simulink model "SWC_HALOUT_type"  (R2021b)
settings: Solver=FixedStepDiscrete  StartTime=0.0  StopTime=10.0  FixedStep=0.005  RelTol=1e-3
undefined symbols (not defined in the file): DIDLen_APPD, DIDLen_APPE, DIDLen_APPPedalZP, DIDLen_APSFunConfig, DIDLen_AutoLock, DIDLen_AutoWipHSpdEN, DIDLen_CALID, DIDLen_CDEODT, DIDLen_CLRDIST, DIDLen_DKCBLESta, DIDLen_DKCKey, DIDLen_DKCSta, DIDLen_DoorNFCAnchorSta, DIDLen_DRLDis, DIDLen_DynoMode, DIDLen_ECUNAME, DIDLen_FDDKCCoordXY, DIDLen_FMHTimer, DIDLen_LFLowPresThre, DIDLen_LFSensorID, DIDLen_LIDAAnchorSta, DIDLen_LRLowPresThre, DIDLen_LRSensorID, DIDLen_MILDIST, DIDLen_NUMPSATRIPSFLTMEMCLR, DIDLen_NVMPedalZP, DIDLen_OBDReq, DIDLen_ODOMETER, DIDLen_PKE, DIDLen_ProtocolId, DIDLen_PSA, DIDLen_QTYPSATRIPS, DIDLen_RFLowPresThre, DIDLen_RFSensorID, DIDLen_RRLowPresThre, DIDLen_RRSensorID, DIDLen_RUNTM, DIDLen_SensorMode, DIDLen_TestGroup, DIDLen_TireSize, DIDLen_TPMSLearnSta, DIDLen_TurnLampFLThreCurr, DIDLen_TurnLampFRThreCurr, DIDLen_TurnLampRLThreCurr, DIDLen_TurnLampRRThreCurr, DIDLen_UIDSta, DIDLen_USSConfig, DIDLen_UWBAnchorSta, DIDLen_VIN, DIDLen_VSS, DIDLen_WhlPres, DIDLen_WhlSensorBattSta, DIDLen_WhlTmp, DIDLen_WipRLSCmdCutFilter, DIDLen_WipRLSCmdHoldFilter, DIDLen_XWDMode, DIDNum_APPD, DIDNum_APPE, DIDNum_APPPedalZP, DIDNum_APSFunConfig ... (+504)
libraries: simulink x893, FVT_lib x320, hdlsllib x6, hcu_lib x5, halout x1
(part 1 of 11)
settings Model: DataDictionary=APPTypes.sldd  Creator=FVT23010  LastModifiedBy=FVT23033
settings DataIOCC: SaveFormat=StructureWithTime
settings OptimizationCC: DefaultParameterBehavior=Inlined  EnhancedBackFolding=on  PassReuseOutputArgsAs=Individual arguments  ZeroExternalMemoryAtStartup=off  ZeroInternalMemoryAtStartup=off  OptimizeBlockOrder=speed  DifferentSizesBufferReuse=on  OptimizationCustomize=off  EfficientTunableParamExpr=on
settings DebuggingCC: ParameterTunabilityLossMsg=error
settings HardwareCC: ProdBitPerPointer=32  ProdBitPerSizeT=32  ProdBitPerPtrDiffT=32  ProdLargestAtomicInteger=Long  ProdLargestAtomicFloat=Double  ProdWordSize=32  ProdLongLongMode=on  ProdHWDeviceType=ARM Compatible->ARM Cortex-M
settings ModelReferenceCC: ModelReferenceNumInstancesAllowed=Single
settings SFSimCC: MATLABDynamicMemAlloc=off
settings RTWCC: Description=AUTOSAR  SystemTargetFile=autosar.tlc  GenCodeOnly=on  TemplateMakefile=ert_default_tmf  PortableWordSizes=on
settings CodeAppCC: ForceParamTrailComments=on  IgnoreCustomStorageClasses=off  OperatorAnnotations=on  SimulinkDataObjDesc=on  SFDataObjDesc=on  InsertBlockDesc=on
settings STFCustomTargetCC: TargetLangStandard=C99 (ISO)  UtilityFuncGeneration=Shared location  MultiwordLength=256  ParMdlRefBuildCompliant=on  CompOptLevelCompliant=on  IncludeMdlTerminateFcn=off  CombineOutputUpdateFcns=on  SuppressErrorStatus=on  ERTCustomFileBanners=on  SupportNonFinite=off  SupportComplex=off  SupportContinuousTime=off  SupportNonInlinedSFcns=off  RemoveResetFunc=on  MATLABClassNameForMDSCustomization=Simulink.SoftwareTarget.ERTCustomization  AutosarCompliant=on  GRTInterface=off  UseToolchainInfoCompliant=on  GenerateSharedConstants=off  LookupTableObjectStructAxisOrder=2,1,3,4,...  LUTObjectStructOrderEvenSpacing=Size,Table,Breakpoints  SystemTargetFile=autosar.tlc
settings ERTTargetCC: TargetLangStandard=C99 (ISO)  UtilityFuncGeneration=Shared location  ConcurrentExecutionCompliant=off  IncludeMdlTerminateFcn=off  SuppressErrorStatus=on  SupportNonFinite=off  SupportComplex=off  ModelStepFunctionPrototypeControlCompliant=off  CPPClassGenCompliant=off  AutosarCompliant=on  GenerateSharedConstants=off  LookupTableObjectStructAxisOrder=2,1,3,4,...  LUTObjectStructOrderEvenSpacing=Size,Table,Breakpoints  GenerateASAP2=on  InlinedParameterPlacement=NonHierarchical  ERTCustomFileTemplate=example_file_process.tlc  ConvertIfToSwitch=off  SuppressUnreachableDefaultCases=off  BooleanTrueId=true_MatlabRTW  BooleanFalseId=false_MatlabRTW

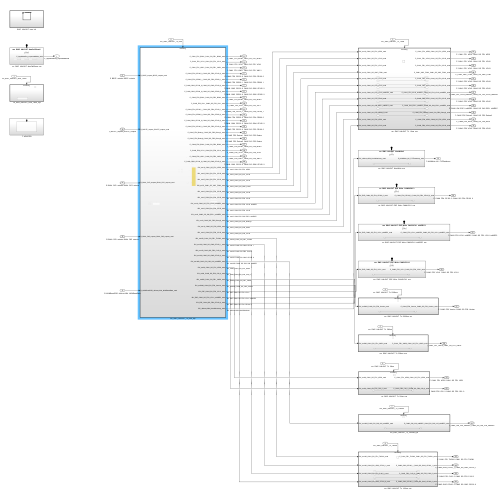
[thumbnail: Simulink's stored preview of the top-level diagram]
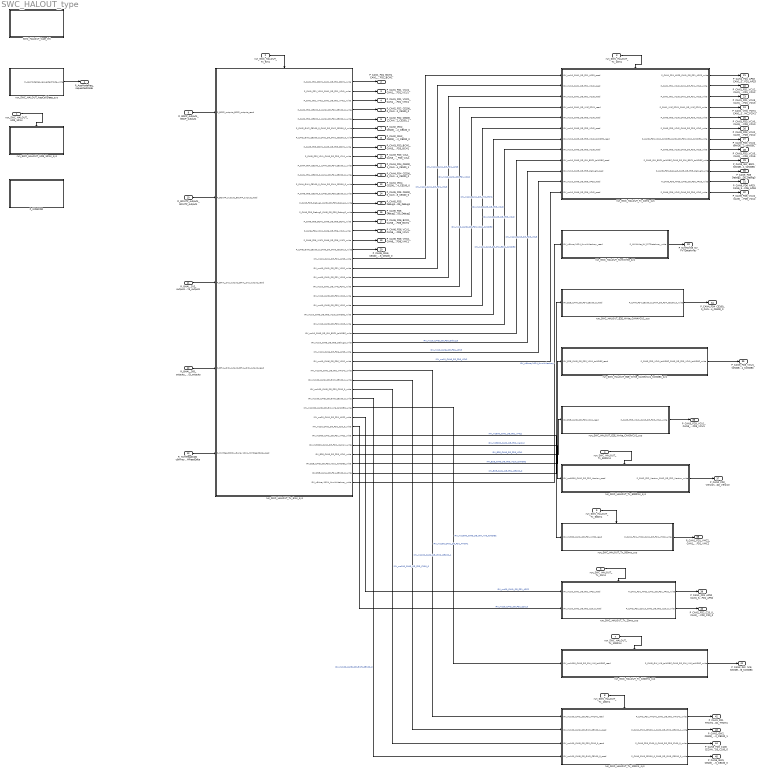
== system SWC_HALOUT_type ==
  run_SWC_HALOUT_UDS_10ms : Inport  SampleTime=0.01  OutputFunctionCall=on
  run_SWC_HALOUT_Tx_5ms : Inport  Port=2  SampleTime=0.005  OutputFunctionCall=on
  run_SWC_HALOUT_Tx_10ms : Inport  Port=3  SampleTime=0.01  OutputFunctionCall=on
  run_SWC_HALOUT_Tx_5000ms : Inport  Port=4  SampleTime=5  OutputFunctionCall=on
  run_SWC_HALOUT_Tx_500ms : Inport  Port=5  SampleTime=0.5  OutputFunctionCall=on
  run_SWC_HALOUT_Tx_20ms : Inport  Port=6  SampleTime=0.02  OutputFunctionCall=on
  run_SWC_HALOUT_Tx_1000ms : Inport  Port=7  SampleTime=1  OutputFunctionCall=on
  run_SWC_HALOUT_Tx_100ms : Inport  Port=8  SampleTime=0.1  OutputFunctionCall=on
  R_BSCP_outputs_BSCP_outputs : Inport  Port=9  OutDataTypeStr=Bus: BSCP_outputs  PortDimensions=1  BusOutputAsStruct=on
  R_BOUTP_outputs_BOUTP_outputs : Inport  Port=10  OutDataTypeStr=Bus: BOUTP_outputs  PortDimensions=1  BusOutputAsStruct=on
  R_BHAL_SYS_outputs_BHAL_SYS_outputs : Inport  Port=11  OutDataTypeStr=Bus: BHAL_SYS_outputs  PortDimensions=1  BusOutputAsStruct=on
  R_BHAL_DID_outputs_BHAL_DID_outputs : Inport  Port=12  OutDataTypeStr=Bus: BHAL_DID_outputs  PortDimensions=1  BusOutputAsStruct=on
  R_NVMReadCDD_u8Array1024_NVMReadData : Inport  Port=13  OutDataTypeStr=uint8  PortDimensions=1024
  P_WDGCDD : Subsystem
  SWC_HALOUT_type_Init : Subsystem
  run_SWC_HALOUT_AppCallSleep_sys : Subsystem
  run_SWC_HALOUT_E2E_Write_CAN3VCU1_sys : Subsystem
  run_SWC_HALOUT_E2E_Write_CAN3VCU1_toNIDEC_sys : Subsystem
  run_SWC_HALOUT_E2E_Write_CAN4VCU1_sys : Subsystem
  run_SWC_HALOUT_NvmWrite_sys : Subsystem
  run_SWC_HALOUT_Tx_1000ms_sys : Subsystem
  run_SWC_HALOUT_Tx_100ms_sys : Subsystem
  run_SWC_HALOUT_Tx_10ms_sys : Subsystem
  run_SWC_HALOUT_Tx_20ms_sys : Subsystem
  run_SWC_HALOUT_Tx_5000ms_sys : Subsystem
  run_SWC_HALOUT_Tx_500ms_sys : Subsystem
  run_SWC_HALOUT_Tx_5ms_sys : Subsystem
  run_SWC_HALOUT_UDS_10ms_sys : Subsystem
  P_AppModeReq_requestedMode : Outport  OutDataTypeStr=Enum: AppModeRequestType  PortDimensions=1
  P_CAN1_FD1_BCM1_CAN1_SG_FD1_BCM1 : Outport  Port=2  OutDataTypeStr=Bus: DT_CAN1_SG_FD1_BCM1  PortDimensions=1  BusOutputAsStruct=on
  P_CAN1_FD1_VCU1_CAN1_SG_FD1_VCU1 : Outport  Port=3  OutDataTypeStr=Bus: DT_CAN1_SG_FD1_VCU1  PortDimensions=1  BusOutputAsStruct=on
  P_CAN1_FD1_VMC1_CAN1_SG_FD1_VMC1 : Outport  Port=4  OutDataTypeStr=Bus: DT_CAN1_SG_FD1_VMC1  PortDimensions=1  BusOutputAsStruct=on
  P_CAN2_FD2_CE100_0_CAN2_SG_FD2_CE100_0 : Outport  Port=5  OutDataTypeStr=Bus: DT_CAN2_SG_FD2_CE100_0  PortDimensions=1  BusOutputAsStruct=on
  P_CAN2_FD2_CE200_1_CAN2_SG_FD2_CE200_1 : Outport  Port=6  OutDataTypeStr=Bus: DT_CAN2_SG_FD2_CE200_1  PortDimensions=1  BusOutputAsStruct=on
  P_CAN2_GW2_CE100_0_CAN2_SG_GW2_CE100_0 : Outport  Port=7  OutDataTypeStr=Bus: DT_CAN2_SG_GW2_CE100_0  PortDimensions=1  BusOutputAsStruct=on
  P_CAN2_GW2_CE200_0_CAN2_SG_GW2_CE200_0 : Outport  Port=8  OutDataTypeStr=Bus: DT_CAN2_SG_GW2_CE200_0  PortDimensions=1  BusOutputAsStruct=on
  P_CAN3_FD3_BCM1_CAN3_SG_FD3_BCM1 : Outport  Port=9  OutDataTypeStr=Bus: DT_CAN3_SG_FD3_BCM1  PortDimensions=1  BusOutputAsStruct=on
  P_CAN3_FD3_V2L1_CAN3_SG_FD3_V2L1 : Outport  Port=10  OutDataTypeStr=Bus: DT_CAN3_SG_FD3_V2L1  PortDimensions=1  BusOutputAsStruct=on
  P_CAN4_FD4_CE100_1_CAN4_SG_FD4_CE100_1 : Outport  Port=11  OutDataTypeStr=Bus: DT_CAN4_SG_FD4_CE100_1  PortDimensions=1  BusOutputAsStruct=on
  P_CAN4_FD4_CE200_0_CAN4_SG_FD4_CE200_0 : Outport  Port=12  OutDataTypeStr=Bus: DT_CAN4_SG_FD4_CE200_0  PortDimensions=1  BusOutputAsStruct=on
  P_CAN4_GW4_CE100_0_CAN4_SG_GW4_CE100_0 : Outport  Port=13  OutDataTypeStr=Bus: DT_CAN4_SG_GW4_CE100_0  PortDimensions=1  BusOutputAsStruct=on
  P_CAN5_FD5_CE100_0_CAN5_SG_FD5_CE100_0 : Outport  Port=14  OutDataTypeStr=Bus: DT_CAN5_SG_FD5_CE100_0  PortDimensions=1  BusOutputAsStruct=on
  P_CAN5_FD5_Debug1_CAN5_SG_FD5_Debug1 : Outport  Port=15  OutDataTypeStr=Bus: DT_CAN5_SG_FD5_Debug1  PortDimensions=1  BusOutputAsStruct=on
  P_CAN5_FD5_Debug2_CAN5_SG_FD5_Debug2 : Outport  Port=16  OutDataTypeStr=Bus: DT_CAN5_SG_FD5_Debug2  PortDimensions=1  BusOutputAsStruct=on
  P_CAN6_FD6_BCM1_CAN6_SG_FD6_BCM1 : Outport  Port=17  OutDataTypeStr=Bus: DT_CAN6_SG_FD6_BCM1  PortDimensions=1  BusOutputAsStruct=on
  P_CAN6_FD6_VCU1_CAN6_SG_FD6_VCU1 : Outport  Port=18  OutDataTypeStr=Bus: DT_CAN6_SG_FD6_VCU1  PortDimensions=1  BusOutputAsStruct=on
  P_CAN6_FD6_VMC1_CAN6_SG_FD6_VMC1 : Outport  Port=19  OutDataTypeStr=Bus: DT_CAN6_SG_FD6_VMC1  PortDimensions=1  BusOutputAsStruct=on
  P_CAN6_GW6_CE100_0_CAN6_SG_GW6_CE100_0 : Outport  Port=20  OutDataTypeStr=Bus: DT_CAN6_SG_GW6_CE100_0  PortDimensions=1  BusOutputAsStruct=on
  P_CAN1_FD1_APS3_CAN1_SG_FD1_APS3 : Outport  Port=21  OutDataTypeStr=Bus: DT_CAN1_SG_FD1_APS3  PortDimensions=1  BusOutputAsStruct=on
  P_CAN1_FD1_VCU2_CAN1_SG_FD1_VCU2 : Outport  Port=22  OutDataTypeStr=Bus: DT_CAN1_SG_FD1_VCU2  PortDimensions=1  BusOutputAsStruct=on
  P_CAN1_FD1_VCU3_CAN1_SG_FD1_VCU3 : Outport  Port=23  OutDataTypeStr=Bus: DT_CAN1_SG_FD1_VCU3  PortDimensions=1  BusOutputAsStruct=on
  P_CAN1_VMC_FCM1_CAN1_SG_VMC_FCM1 : Outport  Port=24  OutDataTypeStr=Bus: DT_CAN1_SG_VMC_FCM1  PortDimensions=1  BusOutputAsStruct=on
  P_CAN3_FD3_VCU0_CAN3_SG_FD3_VCU0 : Outport  Port=25  OutDataTypeStr=Bus: DT_CAN3_SG_FD3_VCU0  PortDimensions=1  BusOutputAsStruct=on
  P_CAN3_FD3_VCU2_CAN3_SG_FD3_VCU2 : Outport  Port=26  OutDataTypeStr=Bus: DT_CAN3_SG_FD3_VCU2  PortDimensions=1  BusOutputAsStruct=on
  P_CAN3_FD3_VCU2_toNIDEC_CAN3_SG_FD3_VCU2_toNIDEC : Outport  Port=27  OutDataTypeStr=Bus: DT_CAN3_SG_FD3_VCU2_toNIDEC  PortDimensions=1  BusOutputAsStruct=on
  P_CAN3_FD3_VCU5_CAN3_SG_FD3_VCU5 : Outport  Port=28  OutDataTypeStr=Bus: DT_CAN3_SG_FD3_VCU5  PortDimensions=1  BusOutputAsStruct=on
  P_CAN3_GW_ESC1_toNIDEC_CAN3_SG_GW_ESC1_toNIDEC : Outport  Port=29  OutDataTypeStr=Bus: DT_CAN3_SG_GW_ESC1_toNIDEC  PortDimensions=1  BusOutputAsStruct=on
  P_CAN5_FD5_Debug3_CAN5_SG_FD5_Debug3 : Outport  Port=30  OutDataTypeStr=Bus: DT_CAN5_SG_FD5_Debug3  PortDimensions=1  BusOutputAsStruct=on
  P_CAN6_FD6_APS3_CAN6_SG_FD6_APS3 : Outport  Port=31  OutDataTypeStr=Bus: DT_CAN6_SG_FD6_APS3  PortDimensions=1  BusOutputAsStruct=on
  P_CAN6_FD6_VCU2_CAN6_SG_FD6_VCU2 : Outport  Port=32  OutDataTypeStr=Bus: DT_CAN6_SG_FD6_VCU2  PortDimensions=1  BusOutputAsStruct=on
  P_NVMWrite_NV_FVTDataArray : Outport  Port=33  OutDataTypeStr=uint8  PortDimensions=1024
  P_CAN4_FD4_CE100_0_CAN4_SG_FD4_CE100_0 : Outport  Port=34  OutDataTypeStr=Bus: DT_CAN4_SG_FD4_CE100_0  PortDimensions=1  BusOutputAsStruct=on
  P_CAN3_FD3_VCU1_toNIDEC_CAN3_SG_FD3_VCU1_toNIDEC : Outport  Port=35  OutDataTypeStr=Bus: DT_CAN3_SG_FD3_VCU1_toNIDEC  PortDimensions=1  BusOutputAsStruct=on
  P_CAN3_FD3_VCU1_CAN3_SG_FD3_VCU1 : Outport  Port=36  OutDataTypeStr=Bus: DT_CAN3_SG_FD3_VCU1  PortDimensions=1  BusOutputAsStruct=on
  P_CAN2_FD2_Version_CAN2_SG_FD2_Version : Outport  Port=37  OutDataTypeStr=Bus: DT_CAN2_SG_FD2_Version  PortDimensions=1  BusOutputAsStruct=on
  P_CAN1_FD1_VMC2_CAN1_SG_FD1_VMC2 : Outport  Port=38  OutDataTypeStr=Bus: DT_CAN1_SG_FD1_VMC2  PortDimensions=1  BusOutputAsStruct=on
  P_CAN1_FD1_APS2_CAN1_SG_FD1_APS2 : Outport  Port=39  OutDataTypeStr=Bus: DT_CAN1_SG_FD1_APS2  PortDimensions=1  BusOutputAsStruct=on
  P_CAN2_FD2_C20_0_CAN2_SG_FD2_C20_0 : Outport  Port=40  OutDataTypeStr=Bus: DT_CAN2_SG_FD2_C20_0  PortDimensions=1  BusOutputAsStruct=on
  P_CAN3_GW_IVI6_toNIDEC_CAN3_SG_GW_IVI6_toNIDEC : Outport  Port=41  OutDataTypeStr=Bus: DT_CAN3_SG_GW_IVI6_toNIDEC  PortDimensions=1  BusOutputAsStruct=on
  P_CAN1_FD1_THCM1_CAN1_SG_FD1_THCM1 : Outport  Port=42  OutDataTypeStr=Bus: DT_CAN1_SG_FD1_THCM1  PortDimensions=1  BusOutputAsStruct=on
  P_CAN2_GW2_CE100_1_CAN2_SG_GW2_CE100_1 : Outport  Port=43  OutDataTypeStr=Bus: DT_CAN2_SG_GW2_CE100_1  PortDimensions=1  BusOutputAsStruct=on
  P_CAN3_FD3_C100_0_CAN3_SG_FD3_C100_0 : Outport  Port=44  OutDataTypeStr=Bus: DT_CAN3_SG_FD3_C100_0  PortDimensions=1  BusOutputAsStruct=on
  P_CAN5_GW5_CE100_0_CAN5_SG_GW5_CE100_0 : Outport  Port=45  OutDataTypeStr=Bus: DT_CAN5_SG_GW5_CE100_0  PortDimensions=1  BusOutputAsStruct=on
  wires:
  run_SWC_HALOUT_AppCallSleep_sys/1(P_AppModeReq_requestedMode_write) -> P_AppModeReq_requestedMode/1
  R_BSCP_outputs_BSCP_outputs/1 -> run_SWC_HALOUT_Tx_5ms_sys/1(R_BSCP_outputs_BSCP_outputs_read)
  R_BOUTP_outputs_BOUTP_outputs/1 -> run_SWC_HALOUT_Tx_5ms_sys/2(R_BOUTP_outputs_BOUTP_outputs_read)
  R_BHAL_SYS_outputs_BHAL_SYS_outputs/1 -> run_SWC_HALOUT_Tx_5ms_sys/3(R_BHAL_SYS_outputs_BHAL_SYS_outputs_read)
  R_BHAL_DID_outputs_BHAL_DID_outputs/1 -> run_SWC_HALOUT_Tx_5ms_sys/4(R_BHAL_DID_outputs_BHAL_DID_outputs_read)
  R_NVMReadCDD_u8Array1024_NVMReadData/1 -> run_SWC_HALOUT_Tx_5ms_sys/5(R_NVMReadCDD_u8Array1024_NVMReadData_read)
  run_SWC_HALOUT_Tx_5ms_sys/1(P_CAN1_FD1_BCM1_CAN1_SG_FD1_BCM1_write) -> P_CAN1_FD1_BCM1_CAN1_SG_FD1_BCM1/1
  run_SWC_HALOUT_Tx_5ms_sys/2(P_CAN1_FD1_VCU1_CAN1_SG_FD1_VCU1_write) -> P_CAN1_FD1_VCU1_CAN1_SG_FD1_VCU1/1
  run_SWC_HALOUT_Tx_5ms_sys/3(P_CAN1_FD1_VMC1_CAN1_SG_FD1_VMC1_write) -> P_CAN1_FD1_VMC1_CAN1_SG_FD1_VMC1/1
  run_SWC_HALOUT_Tx_5ms_sys/4(P_CAN2_FD2_CE100_0_CAN2_SG_FD2_CE100_0_write) -> P_CAN2_FD2_CE100_0_CAN2_SG_FD2_CE100_0/1
  run_SWC_HALOUT_Tx_5ms_sys/5(P_CAN2_FD2_CE200_1_CAN2_SG_FD2_CE200_1_write) -> P_CAN2_FD2_CE200_1_CAN2_SG_FD2_CE200_1/1
  run_SWC_HALOUT_Tx_5ms_sys/6(P_CAN2_GW2_CE100_0_CAN2_SG_GW2_CE100_0_write) -> P_CAN2_GW2_CE100_0_CAN2_SG_GW2_CE100_0/1
  run_SWC_HALOUT_Tx_5ms_sys/7(P_CAN2_GW2_CE200_0_CAN2_SG_GW2_CE200_0_write) -> P_CAN2_GW2_CE200_0_CAN2_SG_GW2_CE200_0/1
  run_SWC_HALOUT_Tx_5ms_sys/8(P_CAN3_FD3_BCM1_CAN3_SG_FD3_BCM1_write) -> P_CAN3_FD3_BCM1_CAN3_SG_FD3_BCM1/1
  run_SWC_HALOUT_Tx_5ms_sys/9(P_CAN3_FD3_V2L1_CAN3_SG_FD3_V2L1_write) -> P_CAN3_FD3_V2L1_CAN3_SG_FD3_V2L1/1
  run_SWC_HALOUT_Tx_5ms_sys/10(P_CAN4_FD4_CE100_1_CAN4_SG_FD4_CE100_1_write) -> P_CAN4_FD4_CE100_1_CAN4_SG_FD4_CE100_1/1
  run_SWC_HALOUT_Tx_5ms_sys/11(P_CAN4_FD4_CE200_0_CAN4_SG_FD4_CE200_0_write) -> P_CAN4_FD4_CE200_0_CAN4_SG_FD4_CE200_0/1
  run_SWC_HALOUT_Tx_5ms_sys/12(P_CAN4_GW4_CE100_0_CAN4_SG_GW4_CE100_0_write) -> P_CAN4_GW4_CE100_0_CAN4_SG_GW4_CE100_0/1
  run_SWC_HALOUT_Tx_5ms_sys/13(P_CAN5_FD5_CE100_0_CAN5_SG_FD5_CE100_0_write) -> P_CAN5_FD5_CE100_0_CAN5_SG_FD5_CE100_0/1
  run_SWC_HALOUT_Tx_5ms_sys/14(P_CAN5_FD5_Debug1_CAN5_SG_FD5_Debug1_write) -> P_CAN5_FD5_Debug1_CAN5_SG_FD5_Debug1/1
  run_SWC_HALOUT_Tx_5ms_sys/15(P_CAN5_FD5_Debug2_CAN5_SG_FD5_Debug2_write) -> P_CAN5_FD5_Debug2_CAN5_SG_FD5_Debug2/1
  run_SWC_HALOUT_Tx_5ms_sys/16(P_CAN6_FD6_BCM1_CAN6_SG_FD6_BCM1_write) -> P_CAN6_FD6_BCM1_CAN6_SG_FD6_BCM1/1
  run_SWC_HALOUT_Tx_5ms_sys/17(P_CAN6_FD6_VCU1_CAN6_SG_FD6_VCU1_write) -> P_CAN6_FD6_VCU1_CAN6_SG_FD6_VCU1/1
  run_SWC_HALOUT_Tx_5ms_sys/18(P_CAN6_FD6_VMC1_CAN6_SG_FD6_VMC1_write) -> P_CAN6_FD6_VMC1_CAN6_SG_FD6_VMC1/1
  run_SWC_HALOUT_Tx_5ms_sys/19(P_CAN6_GW6_CE100_0_CAN6_SG_GW6_CE100_0_write) -> P_CAN6_GW6_CE100_0_CAN6_SG_GW6_CE100_0/1
  run_SWC_HALOUT_Tx_10ms_sys/1(P_CAN1_FD1_APS3_CAN1_SG_FD1_APS3_write) -> P_CAN1_FD1_APS3_CAN1_SG_FD1_APS3/1
  run_SWC_HALOUT_Tx_10ms_sys/2(P_CAN1_FD1_VCU2_CAN1_SG_FD1_VCU2_write) -> P_CAN1_FD1_VCU2_CAN1_SG_FD1_VCU2/1
  run_SWC_HALOUT_Tx_10ms_sys/3(P_CAN1_FD1_VCU3_CAN1_SG_FD1_VCU3_write) -> P_CAN1_FD1_VCU3_CAN1_SG_FD1_VCU3/1
  run_SWC_HALOUT_Tx_10ms_sys/4(P_CAN1_VMC_FCM1_CAN1_SG_VMC_FCM1_write) -> P_CAN1_VMC_FCM1_CAN1_SG_VMC_FCM1/1
  run_SWC_HALOUT_Tx_10ms_sys/5(P_CAN3_FD3_VCU0_CAN3_SG_FD3_VCU0_write) -> P_CAN3_FD3_VCU0_CAN3_SG_FD3_VCU0/1
  run_SWC_HALOUT_Tx_10ms_sys/6(P_CAN3_FD3_VCU2_CAN3_SG_FD3_VCU2_write) -> P_CAN3_FD3_VCU2_CAN3_SG_FD3_VCU2/1
  run_SWC_HALOUT_Tx_10ms_sys/7(P_CAN3_FD3_VCU2_toNIDEC_CAN3_SG_FD3_VCU2_toNIDEC_write) -> P_CAN3_FD3_VCU2_toNIDEC_CAN3_SG_FD3_VCU2_toNIDEC/1
  run_SWC_HALOUT_Tx_10ms_sys/8(P_CAN3_FD3_VCU5_CAN3_SG_FD3_VCU5_write) -> P_CAN3_FD3_VCU5_CAN3_SG_FD3_VCU5/1
  run_SWC_HALOUT_Tx_10ms_sys/9(P_CAN3_GW_ESC1_toNIDEC_CAN3_SG_GW_ESC1_toNIDEC_write) -> P_CAN3_GW_ESC1_toNIDEC_CAN3_SG_GW_ESC1_toNIDEC/1
  run_SWC_HALOUT_Tx_10ms_sys/10(P_CAN5_FD5_Debug3_CAN5_SG_FD5_Debug3_write) -> P_CAN5_FD5_Debug3_CAN5_SG_FD5_Debug3/1
  run_SWC_HALOUT_Tx_10ms_sys/11(P_CAN6_FD6_APS3_CAN6_SG_FD6_APS3_write) -> P_CAN6_FD6_APS3_CAN6_SG_FD6_APS3/1
  run_SWC_HALOUT_Tx_10ms_sys/12(P_CAN6_FD6_VCU2_CAN6_SG_FD6_VCU2_write) -> P_CAN6_FD6_VCU2_CAN6_SG_FD6_VCU2/1
  run_SWC_HALOUT_NvmWrite_sys/1(P_NVMWrite_NV_FVTDataArray_write) -> P_NVMWrite_NV_FVTDataArray/1
  run_SWC_HALOUT_E2E_Write_CAN4VCU1_sys/1(P_CAN4_FD4_CE100_0_CAN4_SG_FD4_CE100_0_write) -> P_CAN4_FD4_CE100_0_CAN4_SG_FD4_CE100_0/1
  run_SWC_HALOUT_E2E_Write_CAN3VCU1_toNIDEC_sys/1(P_CAN3_FD3_VCU1_toNIDEC_CAN3_SG_FD3_VCU1_toNIDEC_write) -> P_CAN3_FD3_VCU1_toNIDEC_CAN3_SG_FD3_VCU1_toNIDEC/1
  run_SWC_HALOUT_E2E_Write_CAN3VCU1_sys/1(P_CAN3_FD3_VCU1_CAN3_SG_FD3_VCU1_write) -> P_CAN3_FD3_VCU1_CAN3_SG_FD3_VCU1/1
  run_SWC_HALOUT_Tx_5000ms_sys/1(P_CAN2_FD2_Version_CAN2_SG_FD2_Version_write) -> P_CAN2_FD2_Version_CAN2_SG_FD2_Version/1
  run_SWC_HALOUT_Tx_500ms_sys/1(P_CAN1_FD1_VMC2_CAN1_SG_FD1_VMC2_write) -> P_CAN1_FD1_VMC2_CAN1_SG_FD1_VMC2/1
  run_SWC_HALOUT_Tx_20ms_sys/1(P_CAN1_FD1_APS2_CAN1_SG_FD1_APS2_write) -> P_CAN1_FD1_APS2_CAN1_SG_FD1_APS2/1
  run_SWC_HALOUT_Tx_20ms_sys/2(P_CAN2_FD2_C20_0_CAN2_SG_FD2_C20_0_write) -> P_CAN2_FD2_C20_0_CAN2_SG_FD2_C20_0/1
  run_SWC_HALOUT_Tx_1000ms_sys/1(P_CAN3_GW_IVI6_toNIDEC_CAN3_SG_GW_IVI6_toNIDEC_write) -> P_CAN3_GW_IVI6_toNIDEC_CAN3_SG_GW_IVI6_toNIDEC/1
  run_SWC_HALOUT_Tx_100ms_sys/1(P_CAN1_FD1_THCM1_CAN1_SG_FD1_THCM1_write) -> P_CAN1_FD1_THCM1_CAN1_SG_FD1_THCM1/1
  run_SWC_HALOUT_Tx_100ms_sys/2(P_CAN2_GW2_CE100_1_CAN2_SG_GW2_CE100_1_write) -> P_CAN2_GW2_CE100_1_CAN2_SG_GW2_CE100_1/1
  run_SWC_HALOUT_Tx_100ms_sys/3(P_CAN3_FD3_C100_0_CAN3_SG_FD3_C100_0_write) -> P_CAN3_FD3_C100_0_CAN3_SG_FD3_C100_0/1
  run_SWC_HALOUT_Tx_100ms_sys/4(P_CAN5_GW5_CE100_0_CAN5_SG_GW5_CE100_0_write) -> P_CAN5_GW5_CE100_0_CAN5_SG_GW5_CE100_0/1
  run_SWC_HALOUT_Tx_5ms_sys/20(IRV_ms10_CAN1_SG_FD1_APS3_write) -> run_SWC_HALOUT_Tx_10ms_sys/1(IRV_ms10_CAN1_SG_FD1_APS3_read)  "IRV_ms10_CAN1_SG_FD1_APS3"
  run_SWC_HALOUT_Tx_5ms_sys/21(IRV_ms10_CAN1_SG_FD1_VCU2_write) -> run_SWC_HALOUT_Tx_10ms_sys/2(IRV_ms10_CAN1_SG_FD1_VCU2_read)  "IRV_ms10_CAN1_SG_FD1_VCU2"
  run_SWC_HALOUT_Tx_5ms_sys/22(IRV_ms10_CAN1_SG_FD1_VCU3_write) -> run_SWC_HALOUT_Tx_10ms_sys/3(IRV_ms10_CAN1_SG_FD1_VCU3_read)  "IRV_ms10_CAN1_SG_FD1_VCU3"
  run_SWC_HALOUT_Tx_5ms_sys/23(IRV_ms10_CAN1_SG_VMC_FCM1_write) -> run_SWC_HALOUT_Tx_10ms_sys/4(IRV_ms10_CAN1_SG_VMC_FCM1_read)  "IRV_ms10_CAN1_SG_VMC_FCM1"
  run_SWC_HALOUT_Tx_5ms_sys/24(IRV_ms10_CAN3_SG_FD3_VCU0_write) -> run_SWC_HALOUT_Tx_10ms_sys/5(IRV_ms10_CAN3_SG_FD3_VCU0_read)  "IRV_ms10_CAN3_SG_FD3_VCU0"
  run_SWC_HALOUT_Tx_5ms_sys/25(IRV_ms10_CAN3_SG_FD3_VCU2_write) -> run_SWC_HALOUT_Tx_10ms_sys/6(IRV_ms10_CAN3_SG_FD3_VCU2_read)  "IRV_ms10_CAN3_SG_FD3_VCU2"
  run_SWC_HALOUT_Tx_5ms_sys/26(IRV_ms10_CAN3_SG_FD3_VCU2_toNIDEC_write) -> run_SWC_HALOUT_Tx_10ms_sys/7(IRV_ms10_CAN3_SG_FD3_VCU2_toNIDEC_read)  "IRV_ms10_CAN3_SG_FD3_VCU2_toNIDEC"
  run_SWC_HALOUT_Tx_5ms_sys/27(IRV_ms10_CAN3_SG_FD3_VCU5_write) -> run_SWC_HALOUT_Tx_10ms_sys/8(IRV_ms10_CAN3_SG_FD3_VCU5_read)  "IRV_ms10_CAN3_SG_FD3_VCU5"
  run_SWC_HALOUT_Tx_5ms_sys/28(IRV_ms10_CAN3_SG_GW_ESC1_toNIDEC_write) -> run_SWC_HALOUT_Tx_10ms_sys/9(IRV_ms10_CAN3_SG_GW_ESC1_toNIDEC_read)  "IRV_ms10_CAN3_SG_GW_ESC1_toNIDEC"
  run_SWC_HALOUT_Tx_5ms_sys/29(IRV_ms10_CAN5_SG_FD5_Debug3_write) -> run_SWC_HALOUT_Tx_10ms_sys/10(IRV_ms10_CAN5_SG_FD5_Debug3_read)  "IRV_ms10_CAN5_SG_FD5_Debug3"
  run_SWC_HALOUT_Tx_5ms_sys/30(IRV_ms10_CAN6_SG_FD6_APS3_write) -> run_SWC_HALOUT_Tx_10ms_sys/11(IRV_ms10_CAN6_SG_FD6_APS3_read)  "IRV_ms10_CAN6_SG_FD6_APS3"
  run_SWC_HALOUT_Tx_5ms_sys/31(IRV_ms10_CAN6_SG_FD6_VCU2_write) -> run_SWC_HALOUT_Tx_10ms_sys/12(IRV_ms10_CAN6_SG_FD6_VCU2_read)  "IRV_ms10_CAN6_SG_FD6_VCU2"
  run_SWC_HALOUT_Tx_5ms_sys/32(IRV_ms100_CAN1_SG_FD1_THCM1_write) -> run_SWC_HALOUT_Tx_100ms_sys/1(IRV_ms100_CAN1_SG_FD1_THCM1_read)  "IRV_ms100_CAN1_SG_FD1_THCM1"
  run_SWC_HALOUT_Tx_5ms_sys/33(IRV_ms100_CAN2_SG_GW2_CE100_1_write) -> run_SWC_HALOUT_Tx_100ms_sys/2(IRV_ms100_CAN2_SG_GW2_CE100_1_read)  "IRV_ms100_CAN2_SG_GW2_CE100_1"
  run_SWC_HALOUT_Tx_5ms_sys/34(IRV_ms100_CAN3_SG_FD3_C100_0_write) -> run_SWC_HALOUT_Tx_100ms_sys/3(IRV_ms100_CAN3_SG_FD3_C100_0_read)  "IRV_ms100_CAN3_SG_FD3_C100_0"
  run_SWC_HALOUT_Tx_5ms_sys/35(IRV_ms100_CAN5_SG_GW5_CE100_0_write) -> run_SWC_HALOUT_Tx_100ms_sys/4(IRV_ms100_CAN5_SG_GW5_CE100_0_read)  "IRV_ms100_CAN5_SG_GW5_CE100_0"
  run_SWC_HALOUT_Tx_5ms_sys/36(IRV_ms1000_CAN3_SG_GW_IVI6_toNIDEC_write) -> run_SWC_HALOUT_Tx_1000ms_sys/1(IRV_ms1000_CAN3_SG_GW_IVI6_toNIDEC_read)  "IRV_ms1000_CAN3_SG_GW_IVI6_toNIDEC"
  run_SWC_HALOUT_Tx_5ms_sys/37(IRV_ms20_CAN1_SG_FD1_APS2_write) -> run_SWC_HALOUT_Tx_20ms_sys/1(IRV_ms20_CAN1_SG_FD1_APS2_read)  "IRV_ms20_CAN1_SG_FD1_APS2"
  run_SWC_HALOUT_Tx_5ms_sys/38(IRV_ms20_CAN2_SG_FD2_C20_0_write) -> run_SWC_HALOUT_Tx_20ms_sys/2(IRV_ms20_CAN2_SG_FD2_C20_0_read)  "IRV_ms20_CAN2_SG_FD2_C20_0"
  run_SWC_HALOUT_Tx_5ms_sys/39(IRV_ms500_CAN1_SG_FD1_VMC2_write) -> run_SWC_HALOUT_Tx_500ms_sys/1(IRV_ms500_CAN1_SG_FD1_VMC2_read)  "IRV_ms500_CAN1_SG_FD1_VMC2"
  run_SWC_HALOUT_Tx_5ms_sys/40(IRV_ms5000_CAN2_SG_FD2_Version_write) -> run_SWC_HALOUT_Tx_5000ms_sys/1(IRV_ms5000_CAN2_SG_FD2_Version_read)  "IRV_ms5000_CAN2_SG_FD2_Version"
  run_SWC_HALOUT_Tx_5ms_sys/41(IRV_E2E_CAN3_SG_FD3_VCU1_write) -> run_SWC_HALOUT_E2E_Write_CAN3VCU1_sys/1(IRV_E2E_CAN3_SG_FD3_VCU1_read)  "IRV_E2E_CAN3_SG_FD3_VCU1"
  run_SWC_HALOUT_Tx_5ms_sys/42(IRV_E2E_CAN3_SG_FD3_VCU1_toNIDEC_write) -> run_SWC_HALOUT_E2E_Write_CAN3VCU1_toNIDEC_sys/1(IRV_E2E_CAN3_SG_FD3_VCU1_toNIDEC_read)  "IRV_E2E_CAN3_SG_FD3_VCU1_toNIDEC"
  run_SWC_HALOUT_Tx_5ms_sys/43(IRV_E2E_CAN4_SG_FD4_CE100_0_write) -> run_SWC_HALOUT_E2E_Write_CAN4VCU1_sys/1(IRV_E2E_CAN4_SG_FD4_CE100_0_read)  "IRV_E2E_CAN4_SG_FD4_CE100_0"
  run_SWC_HALOUT_Tx_5ms_sys/44(IRV_u8Array1024_NvmWriteArray_write) -> run_SWC_HALOUT_NvmWrite_sys/1(IRV_u8Array1024_NvmWriteArray_read)  "IRV_u8Array1024_NvmWriteArray"
  run_SWC_HALOUT_UDS_10ms/1 -> run_SWC_HALOUT_UDS_10ms_sys/Trigger
  run_SWC_HALOUT_Tx_5ms/1 -> run_SWC_HALOUT_Tx_5ms_sys/Trigger
  run_SWC_HALOUT_Tx_10ms/1 -> run_SWC_HALOUT_Tx_10ms_sys/Trigger
  run_SWC_HALOUT_Tx_5000ms/1 -> run_SWC_HALOUT_Tx_5000ms_sys/Trigger
  run_SWC_HALOUT_Tx_500ms/1 -> run_SWC_HALOUT_Tx_500ms_sys/Trigger
  run_SWC_HALOUT_Tx_20ms/1 -> run_SWC_HALOUT_Tx_20ms_sys/Trigger
  run_SWC_HALOUT_Tx_1000ms/1 -> run_SWC_HALOUT_Tx_1000ms_sys/Trigger
  run_SWC_HALOUT_Tx_100ms/1 -> run_SWC_HALOUT_Tx_100ms_sys/Trigger

== system SWC_HALOUT_type/P_WDGCDD ==
  run_SWC_HALOUT_AppCallWDG_End_sys : Subsystem

== system SWC_HALOUT_type/SWC_HALOUT_type_Init ==
  Event Listener : EventListener  EventName=reset

== system SWC_HALOUT_type/run_SWC_HALOUT_AppCallSleep_sys ==
  function : TriggerPort  TriggerType=function-call  IsSimulinkFunction=on  FunctionName=run_SWC_HALOUT_AppCallSleep  VariantControl=(inherit)
  Constant : Constant  Value=TRUE
  Data Type Conversion : DataTypeConversion  OutDataTypeStr=Enum: AppModeRequestType
  Data Type Conversion1 : DataTypeConversion  OutDataTypeStr=uint8
  P_AppModeReq_requestedMode_write : Outport
  wires:
  Data Type Conversion/1 -> P_AppModeReq_requestedMode_write/1
  Data Type Conversion1/1 -> Data Type Conversion/1
  Constant/1 -> Data Type Conversion1/1

== system SWC_HALOUT_type/run_SWC_HALOUT_E2E_Write_CAN3VCU1_sys ==
  IRV_E2E_CAN3_SG_FD3_VCU1_read : Inport
  function : TriggerPort  TriggerType=function-call  IsSimulinkFunction=on  FunctionName=run_SWC_HALOUT_E2E_Write_CAN3VCU1  VariantControl=(inherit)
  P_CAN3_FD3_VCU1_CAN3_SG_FD3_VCU1_write : Outport
  wires:
  IRV_E2E_CAN3_SG_FD3_VCU1_read/1 -> P_CAN3_FD3_VCU1_CAN3_SG_FD3_VCU1_write/1

== system SWC_HALOUT_type/run_SWC_HALOUT_E2E_Write_CAN3VCU1_toNIDEC_sys ==
  IRV_E2E_CAN3_SG_FD3_VCU1_toNIDEC_read : Inport
  function : TriggerPort  TriggerType=function-call  IsSimulinkFunction=on  FunctionName=run_SWC_HALOUT_E2E_Write_CAN3VCU1_toNIDEC  VariantControl=(inherit)
  P_CAN3_FD3_VCU1_toNIDEC_CAN3_SG_FD3_VCU1_toNIDEC_write : Outport
  wires:
  IRV_E2E_CAN3_SG_FD3_VCU1_toNIDEC_read/1 -> P_CAN3_FD3_VCU1_toNIDEC_CAN3_SG_FD3_VCU1_toNIDEC_write/1

== system SWC_HALOUT_type/run_SWC_HALOUT_E2E_Write_CAN4VCU1_sys ==
  IRV_E2E_CAN4_SG_FD4_CE100_0_read : Inport
  function : TriggerPort  TriggerType=function-call  IsSimulinkFunction=on  FunctionName=run_SWC_HALOUT_E2E_Write_CAN4VCU1  VariantControl=(inherit)
  P_CAN4_FD4_CE100_0_CAN4_SG_FD4_CE100_0_write : Outport
  wires:
  IRV_E2E_CAN4_SG_FD4_CE100_0_read/1 -> P_CAN4_FD4_CE100_0_CAN4_SG_FD4_CE100_0_write/1

== system SWC_HALOUT_type/run_SWC_HALOUT_NvmWrite_sys ==
  IRV_u8Array1024_NvmWriteArray_read : Inport
  function : TriggerPort  TriggerType=function-call  IsSimulinkFunction=on  FunctionName=run_SWC_HALOUT_NvmWrite  VariantControl=(inherit)
  P_NVMWrite_NV_FVTDataArray_write : Outport
  wires:
  IRV_u8Array1024_NvmWriteArray_read/1 -> P_NVMWrite_NV_FVTDataArray_write/1

== system SWC_HALOUT_type/run_SWC_HALOUT_Tx_1000ms_sys ==
  IRV_ms1000_CAN3_SG_GW_IVI6_toNIDEC_read : Inport
  function : TriggerPort  TriggerType=function-call  VariantControl=(inherit)  SampleTimeType=periodic  SampleTime=-1
  P_CAN3_GW_IVI6_toNIDEC_CAN3_SG_GW_IVI6_toNIDEC_write : Outport
  wires:
  IRV_ms1000_CAN3_SG_GW_IVI6_toNIDEC_read/1 -> P_CAN3_GW_IVI6_toNIDEC_CAN3_SG_GW_IVI6_toNIDEC_write/1

== system SWC_HALOUT_type/run_SWC_HALOUT_Tx_100ms_sys ==
  IRV_ms100_CAN1_SG_FD1_THCM1_read : Inport
  IRV_ms100_CAN2_SG_GW2_CE100_1_read : Inport  Port=2
  IRV_ms100_CAN3_SG_FD3_C100_0_read : Inport  Port=3
  IRV_ms100_CAN5_SG_GW5_CE100_0_read : Inport  Port=4
  function : TriggerPort  TriggerType=function-call  VariantControl=(inherit)  SampleTimeType=periodic  SampleTime=-1
  P_CAN1_FD1_THCM1_CAN1_SG_FD1_THCM1_write : Outport
  P_CAN2_GW2_CE100_1_CAN2_SG_GW2_CE100_1_write : Outport  Port=2
  P_CAN3_FD3_C100_0_CAN3_SG_FD3_C100_0_write : Outport  Port=3
  P_CAN5_GW5_CE100_0_CAN5_SG_GW5_CE100_0_write : Outport  Port=4
  wires:
  IRV_ms100_CAN1_SG_FD1_THCM1_read/1 -> P_CAN1_FD1_THCM1_CAN1_SG_FD1_THCM1_write/1
  IRV_ms100_CAN2_SG_GW2_CE100_1_read/1 -> P_CAN2_GW2_CE100_1_CAN2_SG_GW2_CE100_1_write/1
  IRV_ms100_CAN3_SG_FD3_C100_0_read/1 -> P_CAN3_FD3_C100_0_CAN3_SG_FD3_C100_0_write/1
  IRV_ms100_CAN5_SG_GW5_CE100_0_read/1 -> P_CAN5_GW5_CE100_0_CAN5_SG_GW5_CE100_0_write/1

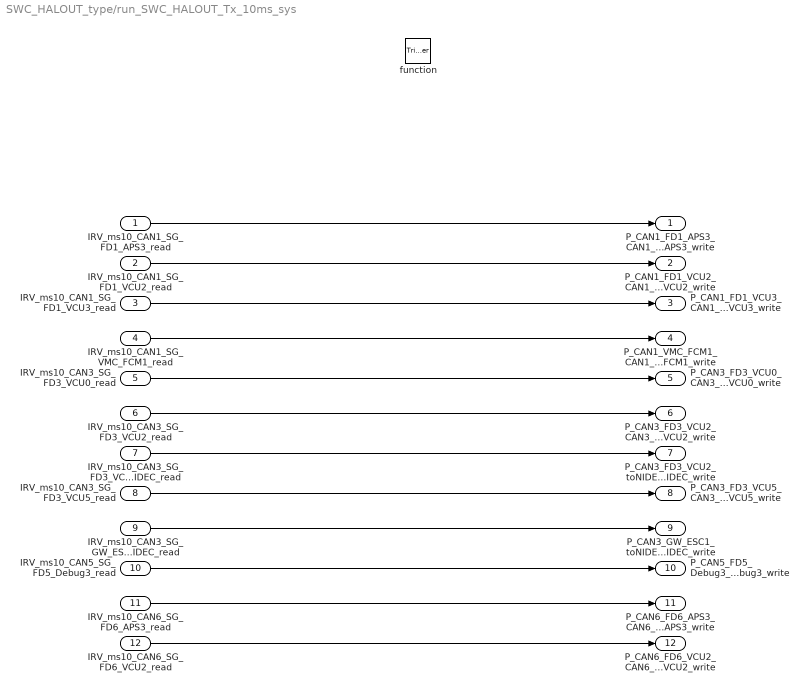
== system SWC_HALOUT_type/run_SWC_HALOUT_Tx_10ms_sys ==
  IRV_ms10_CAN1_SG_FD1_APS3_read : Inport
  IRV_ms10_CAN1_SG_FD1_VCU2_read : Inport  Port=2
  IRV_ms10_CAN1_SG_FD1_VCU3_read : Inport  Port=3
  IRV_ms10_CAN1_SG_VMC_FCM1_read : Inport  Port=4
  IRV_ms10_CAN3_SG_FD3_VCU0_read : Inport  Port=5
  IRV_ms10_CAN3_SG_FD3_VCU2_read : Inport  Port=6
  IRV_ms10_CAN3_SG_FD3_VCU2_toNIDEC_read : Inport  Port=7
  IRV_ms10_CAN3_SG_FD3_VCU5_read : Inport  Port=8
  IRV_ms10_CAN3_SG_GW_ESC1_toNIDEC_read : Inport  Port=9
  IRV_ms10_CAN5_SG_FD5_Debug3_read : Inport  Port=10
  IRV_ms10_CAN6_SG_FD6_APS3_read : Inport  Port=11
  IRV_ms10_CAN6_SG_FD6_VCU2_read : Inport  Port=12
  function : TriggerPort  TriggerType=function-call  VariantControl=(inherit)  SampleTimeType=periodic  SampleTime=-1
  P_CAN1_FD1_APS3_CAN1_SG_FD1_APS3_write : Outport
  P_CAN1_FD1_VCU2_CAN1_SG_FD1_VCU2_write : Outport  Port=2
  P_CAN1_FD1_VCU3_CAN1_SG_FD1_VCU3_write : Outport  Port=3
  P_CAN1_VMC_FCM1_CAN1_SG_VMC_FCM1_write : Outport  Port=4
  P_CAN3_FD3_VCU0_CAN3_SG_FD3_VCU0_write : Outport  Port=5
  P_CAN3_FD3_VCU2_CAN3_SG_FD3_VCU2_write : Outport  Port=6
  P_CAN3_FD3_VCU2_toNIDEC_CAN3_SG_FD3_VCU2_toNIDEC_write : Outport  Port=7
  P_CAN3_FD3_VCU5_CAN3_SG_FD3_VCU5_write : Outport  Port=8
  P_CAN3_GW_ESC1_toNIDEC_CAN3_SG_GW_ESC1_toNIDEC_write : Outport  Port=9
  P_CAN5_FD5_Debug3_CAN5_SG_FD5_Debug3_write : Outport  Port=10
  P_CAN6_FD6_APS3_CAN6_SG_FD6_APS3_write : Outport  Port=11
  P_CAN6_FD6_VCU2_CAN6_SG_FD6_VCU2_write : Outport  Port=12
  wires:
  IRV_ms10_CAN1_SG_FD1_APS3_read/1 -> P_CAN1_FD1_APS3_CAN1_SG_FD1_APS3_write/1
  IRV_ms10_CAN1_SG_FD1_VCU2_read/1 -> P_CAN1_FD1_VCU2_CAN1_SG_FD1_VCU2_write/1
  IRV_ms10_CAN1_SG_FD1_VCU3_read/1 -> P_CAN1_FD1_VCU3_CAN1_SG_FD1_VCU3_write/1
  IRV_ms10_CAN1_SG_VMC_FCM1_read/1 -> P_CAN1_VMC_FCM1_CAN1_SG_VMC_FCM1_write/1
  IRV_ms10_CAN3_SG_FD3_VCU0_read/1 -> P_CAN3_FD3_VCU0_CAN3_SG_FD3_VCU0_write/1
  IRV_ms10_CAN3_SG_FD3_VCU2_read/1 -> P_CAN3_FD3_VCU2_CAN3_SG_FD3_VCU2_write/1
  IRV_ms10_CAN3_SG_FD3_VCU2_toNIDEC_read/1 -> P_CAN3_FD3_VCU2_toNIDEC_CAN3_SG_FD3_VCU2_toNIDEC_write/1
  IRV_ms10_CAN3_SG_FD3_VCU5_read/1 -> P_CAN3_FD3_VCU5_CAN3_SG_FD3_VCU5_write/1
  IRV_ms10_CAN3_SG_GW_ESC1_toNIDEC_read/1 -> P_CAN3_GW_ESC1_toNIDEC_CAN3_SG_GW_ESC1_toNIDEC_write/1
  IRV_ms10_CAN5_SG_FD5_Debug3_read/1 -> P_CAN5_FD5_Debug3_CAN5_SG_FD5_Debug3_write/1
  IRV_ms10_CAN6_SG_FD6_APS3_read/1 -> P_CAN6_FD6_APS3_CAN6_SG_FD6_APS3_write/1
  IRV_ms10_CAN6_SG_FD6_VCU2_read/1 -> P_CAN6_FD6_VCU2_CAN6_SG_FD6_VCU2_write/1

== system SWC_HALOUT_type/run_SWC_HALOUT_Tx_20ms_sys ==
  IRV_ms20_CAN1_SG_FD1_APS2_read : Inport
  IRV_ms20_CAN2_SG_FD2_C20_0_read : Inport  Port=2
  function : TriggerPort  TriggerType=function-call  VariantControl=(inherit)  SampleTimeType=periodic  SampleTime=-1
  P_CAN1_FD1_APS2_CAN1_SG_FD1_APS2_write : Outport
  P_CAN2_FD2_C20_0_CAN2_SG_FD2_C20_0_write : Outport  Port=2
  wires:
  IRV_ms20_CAN1_SG_FD1_APS2_read/1 -> P_CAN1_FD1_APS2_CAN1_SG_FD1_APS2_write/1
  IRV_ms20_CAN2_SG_FD2_C20_0_read/1 -> P_CAN2_FD2_C20_0_CAN2_SG_FD2_C20_0_write/1

== system SWC_HALOUT_type/run_SWC_HALOUT_Tx_5000ms_sys ==
  IRV_ms5000_CAN2_SG_FD2_Version_read : Inport
  function : TriggerPort  TriggerType=function-call  VariantControl=(inherit)  SampleTimeType=periodic  SampleTime=-1
  P_CAN2_FD2_Version_CAN2_SG_FD2_Version_write : Outport
  wires:
  IRV_ms5000_CAN2_SG_FD2_Version_read/1 -> P_CAN2_FD2_Version_CAN2_SG_FD2_Version_write/1

== system SWC_HALOUT_type/run_SWC_HALOUT_Tx_500ms_sys ==
  IRV_ms500_CAN1_SG_FD1_VMC2_read : Inport
  function : TriggerPort  TriggerType=function-call  VariantControl=(inherit)  SampleTimeType=periodic  SampleTime=-1
  P_CAN1_FD1_VMC2_CAN1_SG_FD1_VMC2_write : Outport
  wires:
  IRV_ms500_CAN1_SG_FD1_VMC2_read/1 -> P_CAN1_FD1_VMC2_CAN1_SG_FD1_VMC2_write/1

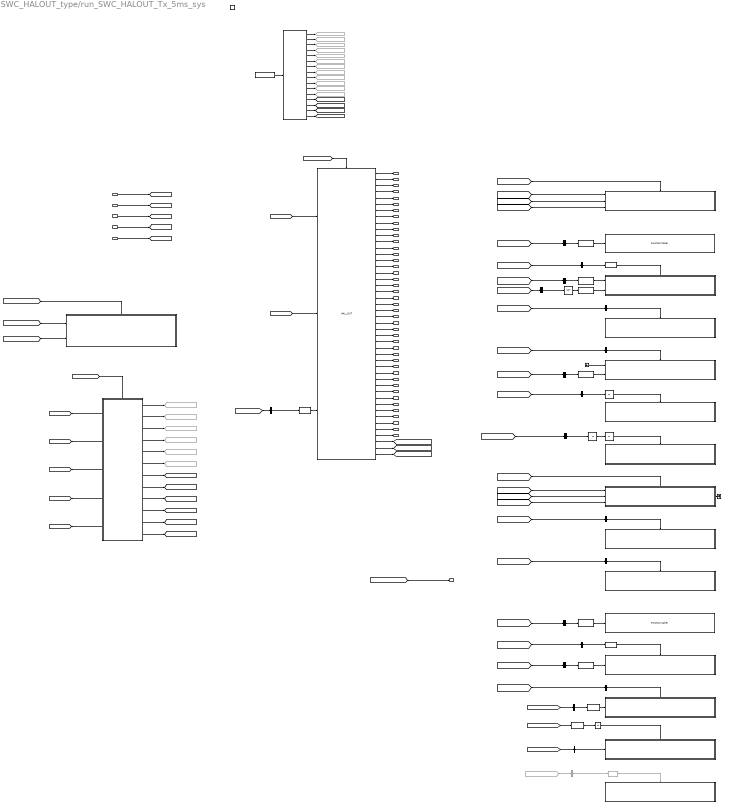
== system SWC_HALOUT_type/run_SWC_HALOUT_Tx_5ms_sys ==
  R_BSCP_outputs_BSCP_outputs_read : Inport
  R_BOUTP_outputs_BOUTP_outputs_read : Inport  Port=2
  R_BHAL_SYS_outputs_BHAL_SYS_outputs_read : Inport  Port=3
  R_BHAL_DID_outputs_BHAL_DID_outputs_read : Inport  Port=4
  R_NVMReadCDD_u8Array1024_NVMReadData_read : Inport  Port=5
  function : TriggerPort  TriggerType=function-call  VariantControl=(inherit)  SampleTimeType=periodic  SampleTime=-1
  Bus Selector15 : BusSelector  OutputSignals=VHAL_AcoreReadyToSlp_flg
  Bus Selector6 : BusSelector  OutputSignals=VHAL_TPMSSensorIDRegResults_raw8
  Bus Selector8 : BusSelector  Commented=on  OutputSignals=VOUTP_ResetPedalZeroPosStart_flg
  Bus Selector9 : BusSelector  OutputSignals=VHAL_DIDSetNVMPedalZP_raw8
  Constant5 : Constant  Value=FALSE
  DIDSet_Subsystem : Subsystem
  Data Type Conversion{,1..2,4..5,107,125} (7 alike) : DataTypeConversion  OutDataTypeStr=uint8
  Data Type Conversion108 : DataTypeConversion  OutDataTypeStr=boolean
  Data Type Conversion3 : DataTypeConversion  OutDataTypeStr=uint32
  Detect Increase1 : simulink/Logic and Bit Operations/Detect Increase  Commented=on  vinit=0.0  OutDataTypeStr=boolean
  From139 : From  Commented=on  GotoTag=BOUTP_outputs
  Goto100 : Goto  Commented=on  GotoTag=trig_Read_NVM_00
  Goto102 : Goto  Commented=on  GotoTag=trig_ReadIMUOffset_00
  Goto105 : Goto  Commented=on  GotoTag=u8_ApsOutSetFrSensorOnCmd
  Goto106 : Goto  Commented=on  GotoTag=trig_GetNMID
  Goto107 : Goto  Commented=on  GotoTag=u8_ApsOutSetFrSensorSwTOCmd
  Goto108 : Goto  Commented=on  GotoTag=u8_ApsOutSetVehSpdTOCmd
  Goto110 : Goto  Commented=on  GotoTag=u8_ApsOutSendChrgPlugSta
  Goto111 : Goto  Commented=on  GotoTag=f32_ApsOutVehSpdSig
  Goto119 : Goto  Commented=on  GotoTag=trig_HAL_DKC_10_3
  Goto122 : Goto  Commented=on  GotoTag=u8_ApsOutGearPosnSig
  Goto90 : Goto  Commented=on  GotoTag=trig_GetDID
  Goto91 : Goto  Commented=on  GotoTag=trig_WDG
  Goto92 : Goto  Commented=on  GotoTag=trig_HAL_DKC_10_2
  Goto93 : Goto  Commented=on  GotoTag=trig_HAL_CDD_10_1
  Goto96 : Goto  Commented=on  GotoTag=trig_OUTP_40
  Goto97 : Goto  Commented=on  GotoTag=trig_APP_30
  Goto98 : Goto  Commented=on  GotoTag=trig_INP_20
  Goto99 : Goto  Commented=on  GotoTag=trig_HAL_IN_10
  Ground10 : Ground
  HALOUT_AFTER : Subsystem
  HAL_OUT : halout/HAL_OUT  SystemSampleTime=-1  VariantActivationTime=update diagram  Latency=0  AutoFrameSizeCalculation=off
  NOT : Logic  Operator=NOT  Inputs=1  AllPortsSameDT=off  OutDataTypeStr=boolean
  OUTP_AFTER : Subsystem
      settings: RTWSystemCode=Nonreusable function  RTWFcnNameOpts=Use subsystem name  RTWFileNameOpts=Use subsystem name
  R_DIDWriteCDD_CSOP_DIDSet_NVMPedalZP : Subsystem
  R_FDCCDD_Inner_CSOP_FDC_AppCallSleep : Subsystem
  R_HALOUTCDD_CSOP_AppNmStateReq : Subsystem
  R_HALOUTCDD_CSOP_ResetPedalZeroPosDone : Subsystem
  R_HALOUTCDD_CSOP_SetAcoreRebootCmdACK : Subsystem
  R_HALOUTCDD_CSOP_SetHazardIND : FunctionCaller  FunctionPrototype=R_HALOUTCDD_CSOP_SetHazardIND(u8_HazardIND)  InputArgumentSpecifications=uint8(1)
  R_HALOUTCDD_CSOP_SetSysPwrStat : FunctionCaller  FunctionPrototype=R_HALOUTCDD_CSOP_SetSysPwrStat(u8_SysPwrStat)  InputArgumentSpecifications=uint8(1)
  R_HALOUTCDD_CSOP_SleepRequest : Subsystem
  R_HALOUTCDD_CSOP_TPMSSensorIDRegSetResults : Subsystem
  R_IOExpOUT_CDD_CSOP_IOExpSetVal : Subsystem
  R_NVMWriteCDD_Inner_NVM_WriteOperation : Subsystem
  R_UDSCDD_CSOP_DdmRestartOperationCycle : Subsystem
  R_UDSCDD_CSOP_SetDTCStatus : Subsystem
  R_WDGCDD_CSOP_Call_WDG_AppEnd : Subsystem
  Terminator_16 : Terminator
  Unit Delay{,1..2,4} (4 alike) : UnitDelay  SampleTime=-1  HasFrameUpgradeWarning=on
  bus_selector : BusSelector  OutputSignals=VOUTP_SysPowerMode_enum
  bus_selector1 : BusSelector  OutputSignals=VOUTP_NetworkReq_flg
  bus_selector10 : BusSelector  OutputSignals=VOUTP_AcoreRebootCmdACK_flg
  bus_selector11 : BusSelector  OutputSignals=VOUTP_HazardIND_flg
  bus_selector12 : BusSelector  OutputSignals=VOUTP_IVIRST_flg
  bus_selector13 : BusSelector  OutputSignals=VOUTP_IVIRST_flg
  bus_selector14 : BusSelector  OutputSignals=VOUTP_TPMSSensorIDRegStart_flg
  bus_selector2 : BusSelector  OutputSignals=VOUTP_NetworkReq_flg
  bus_selector3 : BusSelector  OutputSignals=VOUTP_NetworkReq_flg
  bus_selector4 : BusSelector  OutputSignals=VOUTP_NvWriteReqRisingEdge_flg
  bus_selector5 : BusSelector  OutputSignals=VOUTP_FdcSlpTime_sec
  bus_selector6 : BusSelector  OutputSignals=VOUTP_FdcSlpReqRisingEdge_flg
  bus_selector7 : BusSelector  OutputSignals=VOUTP_FdcSlpReqRisingEdge_flg
  bus_selector8 : BusSelector  OutputSignals=VOUTP_FdcSlpReqRisingEdge_flg
  bus_selector9 : BusSelector  OutputSignals=VOUTP_EnterNewOperCyc_flg
  detect_change : simulink/Logic and Bit Operations/Detect Change  vinit=0  OutDataTypeStr=boolean
  detect_change1 : simulink/Logic and Bit Operations/Detect Change  vinit=0  OutDataTypeStr=boolean
  hcu_main_sched : Stateflow chart  TreatAsAtomicUnit=on
  P_CAN1_FD1_BCM1_CAN1_SG_FD1_BCM1_write : Outport
  P_CAN1_FD1_VCU1_CAN1_SG_FD1_VCU1_write : Outport  Port=2
  P_CAN1_FD1_VMC1_CAN1_SG_FD1_VMC1_write : Outport  Port=3
  P_CAN2_FD2_CE100_0_CAN2_SG_FD2_CE100_0_write : Outport  Port=4
  P_CAN2_FD2_CE200_1_CAN2_SG_FD2_CE200_1_write : Outport  Port=5
  P_CAN2_GW2_CE100_0_CAN2_SG_GW2_CE100_0_write : Outport  Port=6
  P_CAN2_GW2_CE200_0_CAN2_SG_GW2_CE200_0_write : Outport  Port=7
  P_CAN3_FD3_BCM1_CAN3_SG_FD3_BCM1_write : Outport  Port=8
  P_CAN3_FD3_V2L1_CAN3_SG_FD3_V2L1_write : Outport  Port=9
  P_CAN4_FD4_CE100_1_CAN4_SG_FD4_CE100_1_write : Outport  Port=10
  P_CAN4_FD4_CE200_0_CAN4_SG_FD4_CE200_0_write : Outport  Port=11
  P_CAN4_GW4_CE100_0_CAN4_SG_GW4_CE100_0_write : Outport  Port=12
  P_CAN5_FD5_CE100_0_CAN5_SG_FD5_CE100_0_write : Outport  Port=13
  P_CAN5_FD5_Debug1_CAN5_SG_FD5_Debug1_write : Outport  Port=14
  P_CAN5_FD5_Debug2_CAN5_SG_FD5_Debug2_write : Outport  Port=15
  P_CAN6_FD6_BCM1_CAN6_SG_FD6_BCM1_write : Outport  Port=16
  P_CAN6_FD6_VCU1_CAN6_SG_FD6_VCU1_write : Outport  Port=17
  P_CAN6_FD6_VMC1_CAN6_SG_FD6_VMC1_write : Outport  Port=18
  P_CAN6_GW6_CE100_0_CAN6_SG_GW6_CE100_0_write : Outport  Port=19
  IRV_ms10_CAN1_SG_FD1_APS3_write : Outport  Port=20  OutDataTypeStr=Bus: DT_CAN1_SG_FD1_APS3  PortDimensions=1  BusOutputAsStruct=on
  IRV_ms10_CAN1_SG_FD1_VCU2_write : Outport  Port=21  OutDataTypeStr=Bus: DT_CAN1_SG_FD1_VCU2  PortDimensions=1  BusOutputAsStruct=on
  IRV_ms10_CAN1_SG_FD1_VCU3_write : Outport  Port=22  OutDataTypeStr=Bus: DT_CAN1_SG_FD1_VCU3  PortDimensions=1  BusOutputAsStruct=on
  IRV_ms10_CAN1_SG_VMC_FCM1_write : Outport  Port=23  OutDataTypeStr=Bus: DT_CAN1_SG_VMC_FCM1  PortDimensions=1  BusOutputAsStruct=on
  IRV_ms10_CAN3_SG_FD3_VCU0_write : Outport  Port=24  OutDataTypeStr=Bus: DT_CAN3_SG_FD3_VCU0  PortDimensions=1  BusOutputAsStruct=on
  IRV_ms10_CAN3_SG_FD3_VCU2_write : Outport  Port=25  OutDataTypeStr=Bus: DT_CAN3_SG_FD3_VCU2  PortDimensions=1  BusOutputAsStruct=on
  IRV_ms10_CAN3_SG_FD3_VCU2_toNIDEC_write : Outport  Port=26  OutDataTypeStr=Bus: DT_CAN3_SG_FD3_VCU2_toNIDEC  PortDimensions=1  BusOutputAsStruct=on
  IRV_ms10_CAN3_SG_FD3_VCU5_write : Outport  Port=27  OutDataTypeStr=Bus: DT_CAN3_SG_FD3_VCU5  PortDimensions=1  BusOutputAsStruct=on
  IRV_ms10_CAN3_SG_GW_ESC1_toNIDEC_write : Outport  Port=28  OutDataTypeStr=Bus: DT_CAN3_SG_GW_ESC1_toNIDEC  PortDimensions=1  BusOutputAsStruct=on
  IRV_ms10_CAN5_SG_FD5_Debug3_write : Outport  Port=29  OutDataTypeStr=Bus: DT_CAN5_SG_FD5_Debug3  PortDimensions=1  BusOutputAsStruct=on
  IRV_ms10_CAN6_SG_FD6_APS3_write : Outport  Port=30  OutDataTypeStr=Bus: DT_CAN6_SG_FD6_APS3  PortDimensions=1  BusOutputAsStruct=on
  IRV_ms10_CAN6_SG_FD6_VCU2_write : Outport  Port=31  OutDataTypeStr=Bus: DT_CAN6_SG_FD6_VCU2  PortDimensions=1  BusOutputAsStruct=on
  IRV_ms100_CAN1_SG_FD1_THCM1_write : Outport  Port=32  OutDataTypeStr=Bus: DT_CAN1_SG_FD1_THCM1  PortDimensions=1  BusOutputAsStruct=on
  IRV_ms100_CAN2_SG_GW2_CE100_1_write : Outport  Port=33  OutDataTypeStr=Bus: DT_CAN2_SG_GW2_CE100_1  PortDimensions=1  BusOutputAsStruct=on
  IRV_ms100_CAN3_SG_FD3_C100_0_write : Outport  Port=34  OutDataTypeStr=Bus: DT_CAN3_SG_FD3_C100_0  PortDimensions=1  BusOutputAsStruct=on
  IRV_ms100_CAN5_SG_GW5_CE100_0_write : Outport  Port=35  OutDataTypeStr=Bus: DT_CAN5_SG_GW5_CE100_0  PortDimensions=1  BusOutputAsStruct=on
  IRV_ms1000_CAN3_SG_GW_IVI6_toNIDEC_write : Outport  Port=36  OutDataTypeStr=Bus: DT_CAN3_SG_GW_IVI6_toNIDEC  PortDimensions=1  BusOutputAsStruct=on
  IRV_ms20_CAN1_SG_FD1_APS2_write : Outport  Port=37  OutDataTypeStr=Bus: DT_CAN1_SG_FD1_APS2  PortDimensions=1  BusOutputAsStruct=on
  IRV_ms20_CAN2_SG_FD2_C20_0_write : Outport  Port=38  OutDataTypeStr=Bus: DT_CAN2_SG_FD2_C20_0  PortDimensions=1  BusOutputAsStruct=on
  IRV_ms500_CAN1_SG_FD1_VMC2_write : Outport  Port=39  OutDataTypeStr=Bus: DT_CAN1_SG_FD1_VMC2  PortDimensions=1  BusOutputAsStruct=on
  IRV_ms5000_CAN2_SG_FD2_Version_write : Outport  Port=40  OutDataTypeStr=Bus: DT_CAN2_SG_FD2_Version  PortDimensions=1  BusOutputAsStruct=on
  IRV_E2E_CAN3_SG_FD3_VCU1_write : Outport  Port=41  OutDataTypeStr=Bus: DT_CAN3_SG_FD3_VCU1  PortDimensions=1  BusOutputAsStruct=on
  IRV_E2E_CAN3_SG_FD3_VCU1_toNIDEC_write : Outport  Port=42  OutDataTypeStr=Bus: DT_CAN3_SG_FD3_VCU1_toNIDEC  PortDimensions=1  BusOutputAsStruct=on
  IRV_E2E_CAN4_SG_FD4_CE100_0_write : Outport  Port=43  OutDataTypeStr=Bus: DT_CAN4_SG_FD4_CE100_0  PortDimensions=1  BusOutputAsStruct=on
  IRV_u8Array1024_NvmWriteArray_write : Outport  Port=44  OutDataTypeStr=uint8  PortDimensions=1024
  wires:
  [u8Array1024_NvmWriteArray] -> IRV_u8Array1024_NvmWriteArray_write/1
  Data Type Conversion/1 -> R_HALOUTCDD_CSOP_SetSysPwrStat/1
  bus_selector/1 -> Data Type Conversion/1  "<VOUTP_SysPowerMode_enum>"
  [BOUTP_outputs] -> bus_selector/1
  Data Type Conversion1/1 -> R_HALOUTCDD_CSOP_AppNmStateReq/1(WakeReq)
  bus_selector1/1 -> Data Type Conversion1/1  "<VOUTP_NetworkReq_flg>"
  [BOUTP_outputs] -> bus_selector1/1
  Data Type Conversion2/1 -> R_HALOUTCDD_CSOP_AppNmStateReq/2(SleepReq)
  NOT/1 -> Data Type Conversion2/1
  bus_selector2/1 -> NOT/1  "<VOUTP_NetworkReq_flg>"
  [BOUTP_outputs] -> bus_selector2/1
  detect_change/1 -> R_HALOUTCDD_CSOP_AppNmStateReq/Enable
  bus_selector3/1 -> detect_change/1  "<VOUTP_NetworkReq_flg>"
  [BOUTP_outputs] -> bus_selector3/1
  bus_selector4/1 -> R_NVMWriteCDD_Inner_NVM_WriteOperation/Enable  "<VOUTP_NvWriteReqRisingEdge_flg>"
  [BOUTP_outputs] -> bus_selector4/1
  Data Type Conversion3/1 -> R_HALOUTCDD_CSOP_SleepRequest/2(WakeUpTime)
  bus_selector5/1 -> Data Type Conversion3/1  "<VOUTP_FdcSlpTime_sec>"
  [BOUTP_outputs] -> bus_selector5/1
  bus_selector6/1 -> R_HALOUTCDD_CSOP_SleepRequest/Enable  "<VOUTP_FdcSlpReqRisingEdge_flg>"
  [BOUTP_outputs] -> bus_selector6/1
  Unit Delay/1 -> R_WDGCDD_CSOP_Call_WDG_AppEnd/Enable
  bus_selector7/1 -> Unit Delay/1  "<VOUTP_FdcSlpReqRisingEdge_flg>"
  [BOUTP_outputs] -> bus_selector7/1
  Unit Delay1/1 -> R_FDCCDD_Inner_CSOP_FDC_AppCallSleep/Enable
  Unit Delay2/1 -> Unit Delay1/1
  bus_selector8/1 -> Unit Delay2/1  "<VOUTP_FdcSlpReqRisingEdge_flg>"
  [BOUTP_outputs] -> bus_selector8/1
  [Header_Array] -> R_UDSCDD_CSOP_SetDTCStatus/1(Header_Array)
  [DTC_Array] -> R_UDSCDD_CSOP_SetDTCStatus/2(DTC_Array)
  [DTC_Trigger] -> R_UDSCDD_CSOP_SetDTCStatus/Enable
  bus_selector9/1 -> R_UDSCDD_CSOP_DdmRestartOperationCycle/Enable  "<VOUTP_EnterNewOperCyc_flg>"
  [BOUTP_outputs] -> bus_selector9/1
  bus_selector10/1 -> R_HALOUTCDD_CSOP_SetAcoreRebootCmdACK/Enable  "<VOUTP_AcoreRebootCmdACK_flg>"
  [BOUTP_outputs] -> bus_selector10/1
  Data Type Conversion4/1 -> R_HALOUTCDD_CSOP_SetHazardIND/1
  bus_selector11/1 -> Data Type Conversion4/1  "<VOUTP_HazardIND_flg>"
  [BOUTP_outputs] -> bus_selector11/1
  Data Type Conversion5/1 -> R_IOExpOUT_CDD_CSOP_IOExpSetVal/1(In1)
  bus_selector12/1 -> Data Type Conversion5/1  "<VOUTP_IVIRST_flg>"
  [BOUTP_outputs] -> bus_selector12/1
  detect_change1/1 -> R_IOExpOUT_CDD_CSOP_IOExpSetVal/Enable
  bus_selector13/1 -> detect_change1/1  "<VOUTP_IVIRST_flg>"
  [BOUTP_outputs] -> bus_selector13/1
  bus_selector14/1 -> R_HALOUTCDD_CSOP_TPMSSensorIDRegSetResults/Enable  "<VOUTP_TPMSSensorIDRegStart_flg>"
  [BOUTP_outputs] -> bus_selector14/1
  [E2E_CAN3_VCU1_Trigger] -> HALOUT_AFTER/1(E2E_CAN3_VCU1_Trigger)
  [E2E_CAN3_VCU1_toNIDEC_Trigger] -> HALOUT_AFTER/2(E2E_CAN3_VCU1_Trigger_toNIDEC)
  [E2E_CAN4_VCU1_Trigger] -> HALOUT_AFTER/3(E2E_CAN4_VCU1_Trigger)
  [trig_HAL_OUTAFTER_50_1] -> HALOUT_AFTER/Trigger
  [BOUTP_DIDSetData_outputs] -> DIDSet_Subsystem/1(BOUTP_DIDSetData_outputs)
  [BHAL_DID_outputs] -> DIDSet_Subsystem/2(BHAL_DID_outputs)
  [trig_SetDID] -> DIDSet_Subsystem/Trigger
  [BHAL_SYS_outputs] -> Bus Selector15/1
  [trig_HAL_OUT_50] -> HAL_OUT/Trigger
  Bus Selector15/1 -> Data Type Conversion125/1  "<VHAL_AcoreReadyToSlp_flg>"
  [BSCP_outputs] -> HAL_OUT/2
  [BOUTP_outputs] -> HAL_OUT/1
  HAL_OUT/1 -> P_CAN1_FD1_BCM1_CAN1_SG_FD1_BCM1_write/1
  HAL_OUT/2 -> P_CAN1_FD1_VCU1_CAN1_SG_FD1_VCU1_write/1
  HAL_OUT/3 -> P_CAN1_FD1_VMC1_CAN1_SG_FD1_VMC1_write/1
  HAL_OUT/4 -> P_CAN2_FD2_CE100_0_CAN2_SG_FD2_CE100_0_write/1
  HAL_OUT/5 -> P_CAN2_FD2_CE200_1_CAN2_SG_FD2_CE200_1_write/1
  HAL_OUT/6 -> P_CAN2_GW2_CE100_0_CAN2_SG_GW2_CE100_0_write/1
  HAL_OUT/7 -> P_CAN2_GW2_CE200_0_CAN2_SG_GW2_CE200_0_write/1
  HAL_OUT/8 -> P_CAN3_FD3_BCM1_CAN3_SG_FD3_BCM1_write/1
  HAL_OUT/9 -> P_CAN3_FD3_V2L1_CAN3_SG_FD3_V2L1_write/1
  HAL_OUT/10 -> P_CAN4_FD4_CE100_1_CAN4_SG_FD4_CE100_1_write/1
  HAL_OUT/11 -> P_CAN4_FD4_CE200_0_CAN4_SG_FD4_CE200_0_write/1
  HAL_OUT/12 -> P_CAN4_GW4_CE100_0_CAN4_SG_GW4_CE100_0_write/1
  HAL_OUT/13 -> P_CAN5_FD5_CE100_0_CAN5_SG_FD5_CE100_0_write/1
  HAL_OUT/14 -> P_CAN5_FD5_Debug1_CAN5_SG_FD5_Debug1_write/1
  HAL_OUT/15 -> P_CAN5_FD5_Debug2_CAN5_SG_FD5_Debug2_write/1
  HAL_OUT/16 -> P_CAN6_FD6_BCM1_CAN6_SG_FD6_BCM1_write/1
  HAL_OUT/17 -> P_CAN6_FD6_VCU1_CAN6_SG_FD6_VCU1_write/1
  HAL_OUT/18 -> P_CAN6_FD6_VMC1_CAN6_SG_FD6_VMC1_write/1
  HAL_OUT/19 -> P_CAN6_GW6_CE100_0_CAN6_SG_GW6_CE100_0_write/1
  HAL_OUT/20 -> IRV_ms10_CAN1_SG_FD1_APS3_write/1
  HAL_OUT/21 -> IRV_ms10_CAN1_SG_FD1_VCU2_write/1
  HAL_OUT/22 -> IRV_ms10_CAN1_SG_FD1_VCU3_write/1
  HAL_OUT/23 -> IRV_ms10_CAN1_SG_VMC_FCM1_write/1
  HAL_OUT/24 -> IRV_ms10_CAN3_SG_FD3_VCU0_write/1
  HAL_OUT/25 -> IRV_ms10_CAN3_SG_FD3_VCU2_write/1
  HAL_OUT/26 -> IRV_ms10_CAN3_SG_FD3_VCU2_toNIDEC_write/1
  HAL_OUT/27 -> IRV_ms10_CAN3_SG_FD3_VCU5_write/1
  HAL_OUT/28 -> IRV_ms10_CAN3_SG_GW_ESC1_toNIDEC_write/1
  HAL_OUT/29 -> IRV_ms10_CAN5_SG_FD5_Debug3_write/1
  HAL_OUT/30 -> IRV_ms10_CAN6_SG_FD6_APS3_write/1
  HAL_OUT/31 -> IRV_ms10_CAN6_SG_FD6_VCU2_write/1
  HAL_OUT/32 -> IRV_ms100_CAN1_SG_FD1_THCM1_write/1
  HAL_OUT/33 -> IRV_ms100_CAN2_SG_GW2_CE100_1_write/1
  HAL_OUT/34 -> IRV_ms100_CAN3_SG_FD3_C100_0_write/1
  HAL_OUT/35 -> IRV_ms100_CAN5_SG_GW5_CE100_0_write/1
  HAL_OUT/36 -> IRV_ms1000_CAN3_SG_GW_IVI6_toNIDEC_write/1
  HAL_OUT/37 -> IRV_ms20_CAN1_SG_FD1_APS2_write/1
  HAL_OUT/38 -> IRV_ms20_CAN2_SG_FD2_C20_0_write/1
  HAL_OUT/39 -> IRV_ms500_CAN1_SG_FD1_VMC2_write/1
  HAL_OUT/40 -> IRV_ms5000_CAN2_SG_FD2_Version_write/1
  HAL_OUT/41 -> IRV_E2E_CAN3_SG_FD3_VCU1_write/1
  HAL_OUT/42 -> IRV_E2E_CAN3_SG_FD3_VCU1_toNIDEC_write/1
  HAL_OUT/43 -> IRV_E2E_CAN4_SG_FD4_CE100_0_write/1
  HAL_OUT/44 -> [E2E_CAN3_VCU1_Trigger]
  HAL_OUT/45 -> [E2E_CAN3_VCU1_toNIDEC_Trigger]
  HAL_OUT/46 -> [E2E_CAN4_VCU1_Trigger]
  hcu_main_sched/8(trig_HAL_DKC_10_2()) -> Goto92/1
  hcu_main_sched/3(trig_WDG()) -> Goto91/1
  hcu_main_sched/9(trig_HAL_DKC_10_3()) -> Goto119/1
  hcu_main_sched/4(trig_GetNMID()) -> Goto106/1
  hcu_main_sched/15(trig_HAL_OUT_50()) -> [trig_HAL_OUT_50]
  hcu_main_sched/13(trig_OUTP_AFTER_40_1()) -> [trig_OUTP_AFTER_40_1]
  hcu_main_sched/14(trig_SetDID()) -> [trig_SetDID]
  hcu_main_sched/10(trig_INP_20()) -> Goto98/1
  hcu_main_sched/6(trig_HAL_IN_10()) -> Goto99/1
  hcu_main_sched/1(trig_Read_NVM_00()) -> Goto100/1
  hcu_main_sched/5(trig_GetDID()) -> Goto90/1
  hcu_main_sched/16(trig_HAL_OUTAFTER_50_1()) -> [trig_HAL_OUTAFTER_50_1]
  hcu_main_sched/7(trig_HAL_CDD_10_1()) -> Goto93/1
  Constant5/1 -> hcu_main_sched/1(VHAL_FusionSchedReq_flg)
  hcu_main_sched/11(trig_APP_30()) -> Goto97/1
  hcu_main_sched/12(trig_OUTP_40()) -> Goto96/1
  hcu_main_sched/2(trig_ReadIMUOffset_00()) -> Goto102/1
  R_NVMReadCDD_u8Array1024_NVMReadData_read/1 -> [u8Array1024_NvmReadArray]
  R_BSCP_outputs_BSCP_outputs_read/1 -> [BSCP_outputs]
  R_BHAL_DID_outputs_BHAL_DID_outputs_read/1 -> [BHAL_DID_outputs]
  R_BOUTP_outputs_BOUTP_outputs_read/1 -> [BOUTP_outputs]
  R_BHAL_SYS_outputs_BHAL_SYS_outputs_read/1 -> [BHAL_SYS_outputs]
  Ground10/1 -> R_HALOUTCDD_CSOP_SleepRequest/1(SleepState)
  R_UDSCDD_CSOP_SetDTCStatus/1(Out1) -> Terminator_16/1
  [DTC_Constant_Array] -> R_UDSCDD_CSOP_SetDTCStatus/3(In3)
  [BOUTP_DIDSetData_outputs] -> Bus Selector6/1
  Bus Selector6/1 -> Data Type Conversion107/1  "<VHAL_TPMSSensorIDRegResults_raw8>"
  Data Type Conversion107/1 -> R_HALOUTCDD_CSOP_TPMSSensorIDRegSetResults/1(In1)
  Bus Selector9/1 -> R_DIDWriteCDD_CSOP_DIDSet_NVMPedalZP/1(In3)  "<VHAL_DIDSetNVMPedalZP_raw8>"
  [BOUTP_DIDSetData_outputs] -> Bus Selector9/1
  Data Type Conversion108/1 -> Unit Delay4/1
  [u8_ReadPedalZeroPosReq] -> Data Type Conversion108/1
  Unit Delay4/1 -> R_DIDWriteCDD_CSOP_DIDSet_NVMPedalZP/Enable
  Bus Selector8/1 -> Detect Increase1/1  "<VOUTP_ResetPedalZeroPosStart_flg>"
  Detect Increase1/1 -> R_HALOUTCDD_CSOP_ResetPedalZeroPosDone/Enable
  From139/1 -> Bus Selector8/1
  OUTP_AFTER/7(HAL_NvmWriteData_raw) -> [u8Array1024_NvmWriteArray]
  OUTP_AFTER/8(DTC_Trigger) -> [DTC_Trigger]
  [trig_OUTP_AFTER_40_1] -> OUTP_AFTER/Trigger
  OUTP_AFTER/2(ApsOut_SendChrgPlugStaSig) -> Goto110/1
  OUTP_AFTER/11(BOUTP_DIDSetData_outputs) -> [BOUTP_DIDSetData_outputs]
  OUTP_AFTER/3(ApsOut_SetFrSensorOnCmd) -> Goto105/1
  OUTP_AFTER/5(ApsOut_SetVehSpdTOCmd) -> Goto108/1
  OUTP_AFTER/1(ApsOut_GearPosnSig) -> Goto122/1
  OUTP_AFTER/4(ApsOut_SetFrSensorSwTOCmd) -> Goto107/1
  [BHAL_SYS_outputs] -> OUTP_AFTER/2(BHAL_SYSTPMS_outputs)
  [BHAL_SYS_outputs] -> OUTP_AFTER/3(BHAL_SYS_outputs)
  [u8Array1024_NvmReadArray] -> OUTP_AFTER/4(VHAL_NvmReadArray_raw)
  OUTP_AFTER/6(ApsOut_VehSpdSig) -> Goto111/1
  OUTP_AFTER/9(Header_Array) -> [Header_Array]
  [BHAL_DID_outputs] -> OUTP_AFTER/5(BHAL_DIDGetData_raw)
  [BOUTP_outputs] -> OUTP_AFTER/1(BOUTP_outputs)
  OUTP_AFTER/10(DTC_Array) -> [DTC_Array]
  OUTP_AFTER/12(DTC_Constant_Array) -> [DTC_Constant_Array]
  Data Type Conversion125/1 -> HAL_OUT/3

== system SWC_HALOUT_type/run_SWC_HALOUT_UDS_10ms_sys ==
  function : TriggerPort  TriggerType=function-call  VariantControl=(inherit)  SampleTimeType=periodic  SampleTime=-1
  R_HALINCDD_CSOP_UDS_Main : FunctionCaller  FunctionPrototype=R_HALINCDD_CSOP_UDS_Main()

== system SWC_HALOUT_type/P_WDGCDD/run_SWC_HALOUT_AppCallWDG_End_sys ==
  function : TriggerPort  TriggerType=function-call  IsSimulinkFunction=on  FunctionName=run_SWC_HALOUT_AppCallWDG_End  VariantControl=(inherit)
